simulink model "im_with_m1act_damp"  (R2022b)
settings: Solver=FixedStepAuto  StartTime=0.0  StopTime=5  FixedStep=FEM_Ts  MaxStep=FEM_Ts  RelTol=1e-2
InitFcn:
  | %
  | % Initialization callback function
  | %
  | 
  | try
  |    fprintf('\nGMT IMS version (%s)!\n',simulink_fname );
  | 
  |    % Get Simulink model directory
  |    [filepath,name,ext] = fileparts(which(bdroot));
  | 
  |    if ~strcmp(filepath,pwd)
  |       fprintf('\nChanging current directory to \n %s \n',filepath);
  |       cd(filepath);
  |    end
  | 
  |    %
  |  if(osim.bpless_wl)
  |     fprintf('Generating bumpless wind load time series\n');
  |  end
  | catch
  |    warning('Running the InitFcn from puSimulate script');
  | end
values from neighbouring files (symbols this model uses):
  a_max = 250e-6    (= 0.00025)    [load_im_with_m1act_damp.m]    (also in load_m1hp_cpp_demo.m)
  b = B(:,in)*m1sys{seg}.Kbal    [evalM1ofl_act_damp.m]
  c = [Upsilon*C(out0,:);     C(out1a,:)-C(out1b,:);     C(out2,:)]    [evalM1ofl_act_damp.m]
  CS_Upsilon = [0 0 1 3.6925 1.6038 0 0 0 1 0.99769 3.9002 0 ... (1836 elements, 6x306)]    [CS_SupportActuatorArrayConfig.mat]
  delta_sim = 1e-3    (= 0.001)    [load_im_with_m1act_damp.m]    (also in load_m1hp_cpp_demo.m)
  drv_delay = ceil(mount.delay/FEM_Ts)    [load_im_with_m1act_damp.m]    (also in load_m1hp_cpp_demo.m)
  FEM_Ts = 1/1e3    (= 0.001)    [load_im_with_m1act_damp.m]    (also in load_m1hp_cpp_demo.m)
  Hdrive_d = c2d(o.Hdrive(1,1), FEM_Ts, 'tustin')    [load_im_with_m1act_damp.m]    (also in load_m1hp_cpp_demo.m)
  m1_act_lin_d = osim.m1act_damp*1800    [load_im_with_m1act_damp.m]
  m1_act_quad_d = 9000    [load_im_with_m1act_damp.m]
  m1sys = ovr_ofl_crtl(m1sys,seg)    [evalM1ofl_act_damp.m]    (also in load_im_with_m1act_damp.m = ovr_ofl_crtl(m1sys))
  M_cs_abc2xyz = M_cs_abc2xyzT'    [calc_ort2cylTs.m]
  M_oa_abc2xyz = M_oa_abc2xyzT'    [calc_ort2cylTs.m]
  o = fun_confBase(oTest)    [load_im_with_m1act_damp.m]    (also in load_m1hp_cpp_demo.m)
  OA_Upsilon = [1 0 0 0 -0.308856 0.000749419 0 1 0 0.308856 0 0.776768 ... (2010 elements, 6x335)]    [OA_SupportActuatorArrayConfig.mat]
  PG = zeros(length(om2),6)    [load_im_with_m1act_damp.m]    (also in load_m1hp_cpp_demo.m)
  phiB = inputs2ModalF(mode_ind_vec,indDesInputs)    [load_im_with_m1act_damp.m]    (also in load_m1hp_cpp_demo.m)
  phiC = modalDisp2Outputs(indDesOutputs,mode_ind_vec)    [load_im_with_m1act_damp.m]    (also in load_m1hp_cpp_demo.m)
  phiCvel = modalDisp2Outputs(ind_M1act_vel,mode_ind_vec)    [load_im_with_m1act_damp.m]
  Psi_ss = gainMatrix(indDesOutputs,indDesInputs) - K_ss    [load_im_with_m1act_damp.m]    (also in load_m1hp_cpp_demo.m)
  t_gd = 0*0.5    (= 0)    [load_im_with_m1act_damp.m]    (also in load_m1hp_cpp_demo.m)
  t_gd_v = 0*t_gd    (= 0)    [load_im_with_m1act_damp.m]    (also in load_m1hp_cpp_demo.m)
  Tcmd = 12    [load_im_with_m1act_damp.m]    (also in load_m1hp_cpp_demo.m)
  v0 = 0    [load_im_with_m1act_damp.m]    (also in load_m1hp_cpp_demo.m)
  v_max = 50e-6    (= 5e-05)    [load_im_with_m1act_damp.m]    (also in load_m1hp_cpp_demo.m)
  x0 = 0    [load_im_with_m1act_damp.m]    (also in load_m1hp_cpp_demo.m)
  x0_f = xf(end,:)    [load_im_with_m1act_damp.m]    (also in load_m1hp_cpp_demo.m)
undefined symbols (not defined in the file or in its folder): a, A_f, az, az_ff_en, B_f, C_f, D_f, DiscIntNeverNeededParam, el, gir, M_cs_xyz2abc, M_oa_xyz2abc, magnitude, mount, osim
libraries: simulink x9, ims_block_library x7, simulink_extras x2
(part 3 of 3)

== system im_with_m1act_damp/M1 CPP/cmd_pre_proc/Triggered Subsystem/Detect max t_seg ==
  note: initially outputs idx 1
  t_seg : Inport
  Add : Sum  Inputs=+-
  Compare To Zero : simulink/Logic and Bit Operations/Compare To Zero  relop===  OutDataTypeStr=boolean
  For Iterator : ForIterator  ResetStates=reset  IterationSource=external  IterationLimit=3  IndexMode=Zero-based  IterationVariableDataType=int16
  Memory1 : Memory  InitialCondition=int16(1)  InheritSampleTime=on
  MinMax : MinMax  Function=max
  Selector1 : Selector  IndexOptions=Index vector (port)  Indices=[1 3]  OutputSizes=1
  Subtract : Sum  Inputs=+-  OutDataTypeStr=int32  RndMeth=Simplest
  Switch1 : Switch  Criteria=u2 ~= 0  SaturateOnIntegerOverflow=off  InputSameDT=off
  Width1 : Width  DataType=int16
  max_idx : Outport
  max_bool : Outport  Port=2
  wires:
  Width1/1 -> For Iterator/1, Add/1
  Switch1/1 -> Memory1/1, max_idx/1
  For Iterator/1 -> Add/2
  Add/1 -> Switch1/1, Selector1/2  "ii"
  Memory1/1 -> Switch1/3  "idxMinMax"
  Selector1/1 -> Switch1/2  "array(ii)"
  Subtract/1 -> Compare To Zero/1
  t_seg/1 -> Width1/1, MinMax/1, Subtract/1
  MinMax/1 -> Subtract/2
  Compare To Zero/1 -> Selector1/1, max_bool/1

== system im_with_m1act_damp/M1 CPP/cmd_pre_proc/Triggered Subsystem/Detect max t_seg_varsize ==
  t_seg : Inport
  Compare To Zero : simulink/Logic and Bit Operations/Compare To Zero  relop===  OutDataTypeStr=boolean
  Display t_seg : Display  Commented=on
  Find Nonzero Elements : Find  NumberOfInputDimensions=3  OutDataTypeStr=uint8
  Index Vector : MultiPortSwitch  Commented=on  Inputs=1  SaturateOnIntegerOverflow=off  InputSameDT=off
  MinMax : MinMax  Function=max
  MinMax1 : MinMax
  Subtract : Sum  Inputs=+-  OutDataTypeStr=int32  RndMeth=Simplest
  max_idx : Outport
  max_bool : Outport  Port=2
  wires:
  MinMax/1 -> Subtract/2
  Subtract/1 -> Compare To Zero/1
  Find Nonzero Elements/1 -> MinMax1/1
  MinMax1/1 -> max_idx/1, Index Vector/1
  t_seg/1 -> Index Vector/2, Subtract/1, MinMax/1
  Compare To Zero/1 -> max_bool/1, Display t_seg/1, Find Nonzero Elements/1

== system im_with_m1act_damp/M1 CPP/cmd_pre_proc/Triggered Subsystem/Multi-axis demand ==
  x1 : Inport  Partition=on  PartitionDimension=1  PartitionWidth=1  PartitionOffset=0
  x0 : Inport  Port=2  Partition=on  PartitionDimension=1  PartitionWidth=1  PartitionOffset=0
  v1 : Inport  Port=3  Partition=on  PartitionDimension=1  PartitionWidth=1  PartitionOffset=0
  v0 : Inport  Port=4  Partition=on  PartitionDimension=1  PartitionWidth=1  PartitionOffset=0
  Add : Sum
  Add_acd : Sum
  Constant : Constant  Value=a_max
  Constant1 : Constant  Value=v_max
  For Each : ForEach  DisableCoverage=on
  Gain1 : Gain  Gain=1/delta_sim  OutDataTypeStr=uint32
  Gain2 : Gain  Gain=1/delta_sim  OutDataTypeStr=uint32
  Gain3 : Gain  Gain=1/delta_sim  OutDataTypeStr=uint32
  MATLAB Function : MATLAB Function  TreatAsAtomicUnit=on
  t_a : Outport  ConcatenationDimension=1
  t_a_c : Outport  Port=2  ConcatenationDimension=1
  t_a_d : Outport  Port=3  ConcatenationDimension=1
  a_l : Outport  Port=4  ConcatenationDimension=1
  wires:
  x1/1 -> MATLAB Function/1(x1)
  Constant1/1 -> MATLAB Function/3(v_max)
  x0/1 -> MATLAB Function/5(x0)
  v0/1 -> MATLAB Function/6(v0)
  MATLAB Function/4(a_l) -> a_l/1
  Constant/1 -> MATLAB Function/4(a_max)
  v1/1 -> MATLAB Function/2(v1)
  Gain2/1 -> Add/2
  Add/1 -> t_a_c/1, Add_acd/1
  MATLAB Function/2(t_c) -> Gain2/1
  Gain3/1 -> Add_acd/2
  Add_acd/1 -> t_a_d/1
  MATLAB Function/1(t_a) -> Gain1/1
  MATLAB Function/3(t_d) -> Gain3/1
  Gain1/1 -> t_a/1, Add/1

== system im_with_m1act_damp/Mount_Drv_FDR2023_linear/DRV Friction/AZ DT Lugre Fr mode/g(v) ==
  v : Inport
  Enable : EnablePort
  Constant : Constant  Value=0
  Sum : Sum  Inputs=|++
  gc : Constant  Value=Tc/sigma0
  gs : Subsystem
  g : Outport
  wires:
  Constant/1 -> gs/Enable
  gc/1 -> Sum/2
  gs/1(gs(v)) -> Sum/1
  v/1 -> gs/1(v)
  Sum/1 -> g/1

== system im_with_m1act_damp/Mount_Drv_FDR2023_linear/DRV Friction/AZ DT Lugre Fr mode/v2z ==
  v : Inport
  g(v) : Inport  Port=2
  z : Inport  Port=3
  Enable : EnablePort
  Abs : Abs  SaturateOnIntegerOverflow=off
  Divide : Product  Inputs=*/*
  Sum : Sum  Inputs=|+-
  dz : Outport
  wires:
  z/1 -> Divide/3
  g(v)/1 -> Divide/2
  Sum/1 -> dz/1
  v/1 -> Abs/1, Sum/1
  Divide/1 -> Sum/2
  Abs/1 -> Divide/1

== system im_with_m1act_damp/Mount_Drv_FDR2023_linear/DRV Friction/EL DT Lugre Fr model/g(v) ==
  v : Inport
  Enable : EnablePort
  Constant : Constant  Value=0
  Sum : Sum  Inputs=|++
  gc : Constant  Value=Tc/sigma0
  gs : Subsystem
  g : Outport
  wires:
  Constant/1 -> gs/Enable
  gc/1 -> Sum/2
  gs/1(gs(v)) -> Sum/1
  v/1 -> gs/1(v)
  Sum/1 -> g/1

== system im_with_m1act_damp/Mount_Drv_FDR2023_linear/DRV Friction/EL DT Lugre Fr model/v2z ==
  v : Inport
  g(v) : Inport  Port=2
  z : Inport  Port=3
  Enable : EnablePort
  Abs : Abs  SaturateOnIntegerOverflow=off
  Divide : Product  Inputs=*/*
  Sum : Sum  Inputs=|+-
  dz : Outport
  wires:
  z/1 -> Divide/3
  g(v)/1 -> Divide/2
  Sum/1 -> dz/1
  v/1 -> Abs/1, Sum/1
  Divide/1 -> Sum/2
  Abs/1 -> Divide/1

== system im_with_m1act_damp/Mount_Drv_FDR2023_linear/DRV Friction/EL DT Lugre Fr model_/g(v) ==
  v : Inport
  Enable : EnablePort
  Constant : Constant  Value=0
  Sum : Sum  Inputs=|++
  gc : Constant  Value=frParStruct.Tc/frParStruct.sigm0
  gs : Subsystem
  g : Outport  VectorParamsAs1DForOutWhenUnconnected=off
  wires:
  Constant/1 -> gs/Enable
  gc/1 -> Sum/2
  gs/1(gs(v)) -> Sum/1
  v/1 -> gs/1(v)
  Sum/1 -> g/1

== system im_with_m1act_damp/Mount_Drv_FDR2023_linear/DRV Friction/EL DT Lugre Fr model_/v2z ==
  v : Inport
  g(v) : Inport  Port=2
  z : Inport  Port=3
  Enable : EnablePort
  Abs : Abs  SaturateOnIntegerOverflow=off
  Divide : Product  Inputs=*/*
  Sum : Sum  Inputs=|+-
  dz : Outport  VectorParamsAs1DForOutWhenUnconnected=off
  wires:
  z/1 -> Divide/3
  g(v)/1 -> Divide/2
  Sum/1 -> dz/1
  v/1 -> Abs/1, Sum/1
  Divide/1 -> Sum/2
  Abs/1 -> Divide/1

== system im_with_m1act_damp/Mount_Drv_FDR2023_linear/DRV Friction/GIR DT Lugre Fr model/g(v) ==
  v : Inport
  Constant : Constant  Value=0
  Sum : Sum  Inputs=|++
  gc : Constant  Value=Tc/sigma0
  gs : Subsystem
  g : Outport
  wires:
  Constant/1 -> gs/Enable
  gc/1 -> Sum/2
  gs/1(gs(v)) -> Sum/1
  v/1 -> gs/1(v)
  Sum/1 -> g/1

== system im_with_m1act_damp/Mount_Drv_FDR2023_linear/DRV Friction/GIR DT Lugre Fr model/v2z ==
  v : Inport
  g(v) : Inport  Port=2
  z : Inport  Port=3
  Abs : Abs  SaturateOnIntegerOverflow=off
  Divide : Product  Inputs=*/*
  Sum : Sum  Inputs=|+-
  dz : Outport
  wires:
  z/1 -> Divide/3
  g(v)/1 -> Divide/2
  Sum/1 -> dz/1
  v/1 -> Abs/1, Sum/1
  Divide/1 -> Sum/2
  Abs/1 -> Divide/1

== system im_with_m1act_damp/Mount_Drv_FDR2023_linear/DRV Friction/GIR DT Lugre Fr model_/g(v) ==
  v : Inport
  Constant : Constant  Value=0
  Sum : Sum  Inputs=|++
  gc : Constant  Value=frParStruct.Tc/frParStruct.sigm0
  gs : Subsystem
  g : Outport  VectorParamsAs1DForOutWhenUnconnected=off
  wires:
  Constant/1 -> gs/Enable
  gc/1 -> Sum/2
  gs/1(gs(v)) -> Sum/1
  v/1 -> gs/1(v)
  Sum/1 -> g/1

== system im_with_m1act_damp/Mount_Drv_FDR2023_linear/DRV Friction/GIR DT Lugre Fr model_/v2z ==
  note: $\text{Let}\\ |v| = v \sign(v) \\ \text{Sign function approximation:}\\ S_0(v) = \frac{2}{\pi}\atan(k_v v) \\ \text{Then, one approximates the original LuGre model equation}\\ \dot{z} = v - \frac{|v|}{g(v)}z \\ \text{with} \\ \dot{z} = vS_0^2(v) - \frac{vS_0(v)}{g(v)}z .$
  note: Original implementation
  v : Inport
  g(v) : Inport  Port=2
  z : Inport  Port=3
  2/pi : Gain  Gain=2/pi
  Abs1 : Abs  SaturateOnIntegerOverflow=off
  Divide : Product  Inputs=*/*
  Divide1 : Product  Inputs=*/*
  Divide2 : Product  Inputs=**
  Divide3 : Product  Inputs=**
  Math Function : Math  Operator=square  SignedPower=on
  Smoothed-Discontinuous Lugre Model Switch : ManualSwitch
  Sum : Sum  Inputs=|+-
  Sum1 : Sum  Inputs=|+-
  Trigonometric Function : Trigonometry  Operator=atan
  kv : Gain  Gain=1e6%1e-6
  dz : Outport  VectorParamsAs1DForOutWhenUnconnected=off
  wires:
  Smoothed-Discontinuous Lugre Model Switch/1 -> dz/1
  Sum/1 -> Smoothed-Discontinuous Lugre Model Switch/1  "Smoothed Lugre"
  Divide2/1 -> Sum/1
  Divide3/1 -> Divide/1  "S_2"
  Math Function/1 -> Divide2/2  "S_1"
  2/pi/1 -> Math Function/1, Divide3/1  "S_0"
  kv/1 -> Trigonometric Function/1
  Trigonometric Function/1 -> 2/pi/1
  v/1 -> Divide2/1, kv/1, Divide3/2, Sum1/1, Abs1/1
  z/1 -> Divide/3, Divide1/3
  Sum1/1 -> Smoothed-Discontinuous Lugre Model Switch/2  "Discontinuous"
  Abs1/1 -> Divide1/1
  g(v)/1 -> Divide/2, Divide1/2
  Divide1/1 -> Sum1/2
  Divide/1 -> Sum/2

== system im_with_m1act_damp/Mount_Drv_FDR2023_linear/Friction/Friction Alt/g(v) ==
  v : Inport
  Enable : EnablePort
  Constant : Constant  Value=0
  Sum : Sum  Inputs=|++
  gc : Constant  Value=Tc/sigma0
  gs : Subsystem
  g : Outport
  wires:
  Sum/1 -> g/1
  v/1 -> gs/1(v)
  gs/1(gs(v)) -> Sum/1
  gc/1 -> Sum/2
  Constant/1 -> gs/Enable

== system im_with_m1act_damp/Mount_Drv_FDR2023_linear/Friction/Friction Alt/v2z ==
  v : Inport
  g(v) : Inport  Port=2
  z : Inport  Port=3
  Enable : EnablePort
  Abs : Abs  SaturateOnIntegerOverflow=off
  Divide : Product  Inputs=*/*
  Sum : Sum  Inputs=|+-
  dz : Outport
  wires:
  Abs/1 -> Divide/1
  Divide/1 -> Sum/2
  v/1 -> Sum/1, Abs/1
  Sum/1 -> dz/1
  g(v)/1 -> Divide/2
  z/1 -> Divide/3

== system im_with_m1act_damp/Mount_Drv_FDR2023_linear/Friction/Friction Az/g(v) ==
  v : Inport
  Enable : EnablePort
  Constant : Constant  Value=0
  Sum : Sum  Inputs=|++
  gc : Constant  Value=Tc/sigma0
  gs : Subsystem
  g : Outport
  wires:
  Sum/1 -> g/1
  v/1 -> gs/1(v)
  gs/1(gs(v)) -> Sum/1
  gc/1 -> Sum/2
  Constant/1 -> gs/Enable

== system im_with_m1act_damp/Mount_Drv_FDR2023_linear/Friction/Friction Az/v2z ==
  v : Inport
  g(v) : Inport  Port=2
  z : Inport  Port=3
  Enable : EnablePort
  Abs : Abs  SaturateOnIntegerOverflow=off
  Divide : Product  Inputs=*/*
  Sum : Sum  Inputs=|+-
  dz : Outport
  wires:
  Abs/1 -> Divide/1
  Divide/1 -> Sum/2
  v/1 -> Sum/1, Abs/1
  Sum/1 -> dz/1
  g(v)/1 -> Divide/2
  z/1 -> Divide/3

== system im_with_m1act_damp/Mount_Drv_FDR2023_linear/Friction/Friction Gir/PT1 ==
  in : Inport
  Transfer Fcn : TransferFcn  Denominator=[1/(2*pi*f) 1]
  out : Outport
  wires:
  in/1 -> Transfer Fcn/1
  Transfer Fcn/1 -> out/1

== system im_with_m1act_damp/Mount_Drv_FDR2023_linear/Friction/Friction Gir/g(v) ==
  v : Inport
  Constant : Constant  Value=0
  Sum : Sum  Inputs=|++
  gc : Constant  Value=Tc/sigma0
  gs : Subsystem
  g : Outport
  wires:
  Sum/1 -> g/1
  v/1 -> gs/1(v)
  gs/1(gs(v)) -> Sum/1
  gc/1 -> Sum/2
  Constant/1 -> gs/Enable

== system im_with_m1act_damp/Mount_Drv_FDR2023_linear/Friction/Friction Gir/v2z ==
  v : Inport
  g(v) : Inport  Port=2
  z : Inport  Port=3
  Abs : Abs  SaturateOnIntegerOverflow=off
  Divide : Product  Inputs=*/*
  Sum : Sum  Inputs=|+-
  dz : Outport
  wires:
  Abs/1 -> Divide/1
  Divide/1 -> Sum/2
  v/1 -> Sum/1, Abs/1
  Sum/1 -> dz/1
  g(v)/1 -> Divide/2
  z/1 -> Divide/3

== system im_with_m1act_damp/Mount_Drv_FDR2023_linear/Parasitic torque model/Parasitic AZ/For Each Subsystem ==
  In1 : Inport  Partition=on  PartitionDimension=1  PartitionWidth=1  PartitionOffset=0
  EMF Spatial Pattern (N/A) : Sin  TimeSource=Use external signal  Amplitude=oParasitic.oEmf.SpAmp_NPerA  Frequency=oParasitic.oEmf.SpFreq_mmInv*2*pi  Phase=oParasitic.oEmf.SpPhase_rad  SampleTime=0
  For Each : ForEach  DisableCoverage=on
  Sum of Elements2 : Sum  Inputs=+
  Out1 : Outport  ConcatenationDimension=1
  wires:
  Sum of Elements2/1 -> Out1/1
  In1/1 -> EMF Spatial Pattern (N/A)/1
  EMF Spatial Pattern (N/A)/1 -> Sum of Elements2/1

== system im_with_m1act_damp/Mount_Drv_FDR2023_linear/Parasitic torque model/Parasitic AZ/For Each Subsystem1 ==
  In1 : Inport  Partition=on  PartitionDimension=1  PartitionWidth=1  PartitionOffset=0
  Cogging Spatial Pattern (N) : Sin  TimeSource=Use external signal  Amplitude=oParasitic.oCog.SpAmp_N  Frequency=oParasitic.oCog.SpFreq_mmInv*2*pi  Phase=oParasitic.oCog.SpPhase_rad  SampleTime=0
  For Each : ForEach  DisableCoverage=on
  Sum of Elements2 : Sum  Inputs=+
  Out1 : Outport  ConcatenationDimension=1
  wires:
  Sum of Elements2/1 -> Out1/1
  In1/1 -> Cogging Spatial Pattern (N)/1
  Cogging Spatial Pattern (N)/1 -> Sum of Elements2/1

== system im_with_m1act_damp/Mount_Drv_FDR2023_linear/Parasitic torque model/Parasitic EL/For Each Subsystem ==
  In1 : Inport  Partition=on  PartitionDimension=1  PartitionWidth=1  PartitionOffset=0
  EMF Spatial Pattern (N/A) : Sin  TimeSource=Use external signal  Amplitude=oParasitic.oEmf.SpAmp_NPerA  Frequency=oParasitic.oEmf.SpFreq_mmInv*2*pi  Phase=oParasitic.oEmf.SpPhase_rad  SampleTime=0
  For Each : ForEach  DisableCoverage=on
  Sum of Elements2 : Sum  Inputs=+
  Out1 : Outport  ConcatenationDimension=1
  wires:
  Sum of Elements2/1 -> Out1/1
  In1/1 -> EMF Spatial Pattern (N/A)/1
  EMF Spatial Pattern (N/A)/1 -> Sum of Elements2/1

== system im_with_m1act_damp/Mount_Drv_FDR2023_linear/Parasitic torque model/Parasitic EL/For Each Subsystem1 ==
  In1 : Inport  Partition=on  PartitionDimension=1  PartitionWidth=1  PartitionOffset=0
  Cogging Spatial Pattern (N) : Sin  TimeSource=Use external signal  Amplitude=oParasitic.oCog.SpAmp_N  Frequency=oParasitic.oCog.SpFreq_mmInv*2*pi  Phase=oParasitic.oCog.SpPhase_rad  SampleTime=0
  For Each : ForEach  DisableCoverage=on
  Sum of Elements2 : Sum  Inputs=+
  Out1 : Outport  ConcatenationDimension=1
  wires:
  Sum of Elements2/1 -> Out1/1
  In1/1 -> Cogging Spatial Pattern (N)/1
  Cogging Spatial Pattern (N)/1 -> Sum of Elements2/1

== system im_with_m1act_damp/Mount_Drv_FDR2023_linear/Parasitic torque model/Parasitic GIR/For Each Subsystem ==
  In1 : Inport  Partition=on  PartitionDimension=1  PartitionWidth=1  PartitionOffset=0
  (N/A) : Sin  TimeSource=Use external signal  Amplitude=oParasitic.oEmf.SpAmp_NmPerA  Frequency=oParasitic.oEmf.SpFreq_degInv*2*pi  Phase=oParasitic.oEmf.SpPhase_rad  SampleTime=0
  For Each : ForEach  DisableCoverage=on
  Sum of Elements2 : Sum  Inputs=+
  Out1 : Outport  ConcatenationDimension=1
  wires:
  Sum of Elements2/1 -> Out1/1
  In1/1 -> (N/A)/1
  (N/A)/1 -> Sum of Elements2/1

== system im_with_m1act_damp/Mount_Drv_FDR2023_linear/Parasitic torque model/Parasitic GIR/For Each Subsystem1 ==
  In1 : Inport  Partition=on  PartitionDimension=1  PartitionWidth=1  PartitionOffset=0
  Cogging Spatial Pattern (N) : Sin  TimeSource=Use external signal  Amplitude=oParasitic.oCog.SpAmp_Nm  Frequency=oParasitic.oCog.SpFreq_degInv*2*pi  Phase=oParasitic.oCog.SpPhase_rad  SampleTime=0
  For Each : ForEach  DisableCoverage=on
  Sum of Elements2 : Sum  Inputs=+
  Out1 : Outport  ConcatenationDimension=1
  wires:
  Sum of Elements2/1 -> Out1/1
  In1/1 -> Cogging Spatial Pattern (N)/1
  Cogging Spatial Pattern (N)/1 -> Sum of Elements2/1

== system im_with_m1act_damp/Mount_Drv_FDR2023_linear/DRV Friction/AZ DT Lugre Fr mode/g(v)/gs ==
  v : Inport
  Enable : EnablePort
  Divide : Product  Inputs=**
  Gain : Gain  Gain=1/vs
  Math Function : Math  SignedPower=on
  Math Function1 : Math  Operator=magnitude^2  SignedPower=on
  Unary Minus : UnaryMinus
  gs : Constant  Value=(Ts-Tc)/sigma0
  gs(v) : Outport
  wires:
  Divide/1 -> gs(v)/1
  v/1 -> Gain/1
  Gain/1 -> Math Function1/1
  Unary Minus/1 -> Math Function/1
  Math Function1/1 -> Unary Minus/1
  gs/1 -> Divide/2
  Math Function/1 -> Divide/1

== system im_with_m1act_damp/Mount_Drv_FDR2023_linear/DRV Friction/EL DT Lugre Fr model/g(v)/gs ==
  v : Inport
  Enable : EnablePort
  Divide : Product  Inputs=**
  Gain : Gain  Gain=1/vs
  Math Function : Math  SignedPower=on
  Math Function1 : Math  Operator=magnitude^2  SignedPower=on
  Unary Minus : UnaryMinus
  gs : Constant  Value=(Ts-Tc)/sigma0
  gs(v) : Outport
  wires:
  Divide/1 -> gs(v)/1
  v/1 -> Gain/1
  Gain/1 -> Math Function1/1
  Unary Minus/1 -> Math Function/1
  Math Function1/1 -> Unary Minus/1
  gs/1 -> Divide/2
  Math Function/1 -> Divide/1

== system im_with_m1act_damp/Mount_Drv_FDR2023_linear/DRV Friction/EL DT Lugre Fr model_/g(v)/gs ==
  v : Inport
  Enable : EnablePort
  Divide : Product  Inputs=**
  Gain : Gain  Gain=1/frParStruct.vs
  Math Function : Math  SignedPower=on
  Math Function1 : Math  Operator=magnitude^2  SignedPower=on
  Unary Minus : UnaryMinus
  gs : Constant  Value=(frParStruct.Ts-frParStruct.Tc)/frParStruct.sigm0
  gs(v) : Outport  VectorParamsAs1DForOutWhenUnconnected=off
  wires:
  Divide/1 -> gs(v)/1
  v/1 -> Gain/1
  Gain/1 -> Math Function1/1
  Unary Minus/1 -> Math Function/1
  Math Function1/1 -> Unary Minus/1
  gs/1 -> Divide/2
  Math Function/1 -> Divide/1

== system im_with_m1act_damp/Mount_Drv_FDR2023_linear/DRV Friction/GIR DT Lugre Fr model/g(v)/gs ==
  v : Inport
  Enable : EnablePort
  Divide : Product  Inputs=**
  Gain : Gain  Gain=1/vs
  Math Function : Math  SignedPower=on
  Math Function1 : Math  Operator=magnitude^2  SignedPower=on
  Unary Minus : UnaryMinus
  gs : Constant  Value=(Ts-Tc)/sigma0
  gs(v) : Outport
  wires:
  Divide/1 -> gs(v)/1
  v/1 -> Gain/1
  Gain/1 -> Math Function1/1
  Unary Minus/1 -> Math Function/1
  Math Function1/1 -> Unary Minus/1
  gs/1 -> Divide/2
  Math Function/1 -> Divide/1

== system im_with_m1act_damp/Mount_Drv_FDR2023_linear/DRV Friction/GIR DT Lugre Fr model_/g(v)/gs ==
  v : Inport
  Enable : EnablePort
  Divide : Product  Inputs=**
  Gain : Gain  Gain=1/frParStruct.vs
  Math Function : Math  SignedPower=on
  Math Function1 : Math  Operator=magnitude^2  SignedPower=on
  Unary Minus : UnaryMinus
  gs : Constant  Value=(frParStruct.Ts-frParStruct.Tc)/frParStruct.sigm0
  gs(v) : Outport  VectorParamsAs1DForOutWhenUnconnected=off
  wires:
  Divide/1 -> gs(v)/1
  v/1 -> Gain/1
  Gain/1 -> Math Function1/1
  Unary Minus/1 -> Math Function/1
  Math Function1/1 -> Unary Minus/1
  gs/1 -> Divide/2
  Math Function/1 -> Divide/1

== system im_with_m1act_damp/Mount_Drv_FDR2023_linear/Friction/Friction Alt/g(v)/gs ==
  v : Inport
  Enable : EnablePort
  Divide : Product  Inputs=**
  Gain : Gain  Gain=1/vs
  Math Function : Math  SignedPower=on
  Math Function1 : Math  Operator=magnitude^2  SignedPower=on
  Unary Minus : UnaryMinus
  gs : Constant  Value=(Ts-Tc)/sigma0
  gs(v) : Outport
  wires:
  Math Function/1 -> Divide/1
  gs/1 -> Divide/2
  Math Function1/1 -> Unary Minus/1
  Unary Minus/1 -> Math Function/1
  Gain/1 -> Math Function1/1
  v/1 -> Gain/1
  Divide/1 -> gs(v)/1

== system im_with_m1act_damp/Mount_Drv_FDR2023_linear/Friction/Friction Az/g(v)/gs ==
  v : Inport
  Enable : EnablePort
  Divide : Product  Inputs=**
  Gain : Gain  Gain=1/vs
  Math Function : Math  SignedPower=on
  Math Function1 : Math  Operator=magnitude^2  SignedPower=on
  Unary Minus : UnaryMinus
  gs : Constant  Value=(Ts-Tc)/sigma0
  gs(v) : Outport
  wires:
  Math Function/1 -> Divide/1
  gs/1 -> Divide/2
  Math Function1/1 -> Unary Minus/1
  Unary Minus/1 -> Math Function/1
  Gain/1 -> Math Function1/1
  v/1 -> Gain/1
  Divide/1 -> gs(v)/1

== system im_with_m1act_damp/Mount_Drv_FDR2023_linear/Friction/Friction Gir/g(v)/gs ==
  v : Inport
  Enable : EnablePort
  Divide : Product  Inputs=**
  Gain : Gain  Gain=1/vs
  Math Function : Math  SignedPower=on
  Math Function1 : Math  Operator=magnitude^2  SignedPower=on
  Unary Minus : UnaryMinus
  gs : Constant  Value=(Ts-Tc)/sigma0
  gs(v) : Outport
  wires:
  Math Function/1 -> Divide/1
  gs/1 -> Divide/2
  Math Function1/1 -> Unary Minus/1
  Unary Minus/1 -> Math Function/1
  Gain/1 -> Math Function1/1
  v/1 -> Gain/1
  Divide/1 -> gs(v)/1

== matlab function im_with_m1act_damp/M1 CPP/cmd_pre_proc/Triggered Subsystem/Multi-axis demand/MATLAB Function ==
  data: x1 input; t_a output; v1 input; v_max input; a_max input; x0 input; v0 input; t_c output; t_d output; a_l output
%% Calculate duration of each intercept trajectory stage 
%%
function [t_a,t_c,t_d, a_l] = calc_demand(x1, v1, v_max, a_max, x0, v0)

Dv = v1 - v0;
Dx = x1 - x0;

a_l = a_max;
v_l = v_max;
if(Dx < 0)
    a_l = -a_l;
    v_l = -v_l;
end

% Deceleration time
t_d = abs(1/a_l)* sqrt(0.5*(Dv^2) + Dx*a_l);
% Acceleration time
t_a = Dv/a_l + t_d;
if(t_a < 0)
    t_a = 0;
    fprintf("=> t_a=%g, t_d=%g, a_l=%g, D_v=%g\n",t_a, t_d, a_l, Dv);
end

% Check if velocity exceeds the limit at the inflection instant
if( abs(v0+a_l*t_a) > abs(v_l))
    t_a = (1/a_l)* (v_l - v0);
    t_d = (1/a_l)* (v_l - v1);
    t_c = (Dx +Dv*t_a -(v_l-v1)*t_d +0.5*a_l*(t_d^2 - t_a^2)) / (v_l -v1);
else
    t_c = 0;
end

end
